simulink model "Pendulo"  (R2018b)
settings: Solver=ode1  StartTime=0.0  StopTime=100.0  FixedStep=0.5  MaxStep=1e-4  RelTol=1e-3
settings Model: Creator=faraday  LastModifiedBy=alejandro

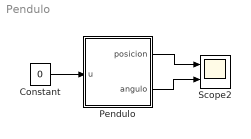
== system Pendulo ==
  Constant : Constant  Value=0
  Pendulo : Subsystem  mask{mc=10, mp=1, l=4, g=9.8, fc=0, fp=0, x10=0, x20=0, x30=pi/2, x40=0}
      mask prompts: mc "masa carro"; mp "masa pendulo"; l "longitud barra"; g "gravedad"; fc "friccion carro"; fp "friccion pendulo"; x10 "posicion inicial"; x20 "velocidad inicial"; x30 "angulo inicial"; x40 "velocidad angular inicial"
  Scope2 : Scope  NumInputPorts=2
  wires:
  Pendulo/1(posicion) -> Scope2/1
  Constant/1 -> Pendulo/1("u ")
  Pendulo/2(angulo) -> Scope2/2

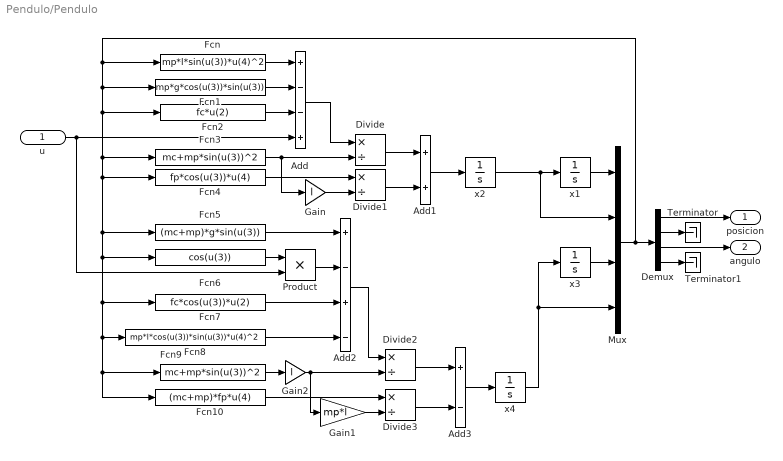
== system Pendulo/Pendulo ==
  "u " : Inport
  Add : Sum  Inputs=+--+
  Add1 : Sum
  Add2 : Sum  Inputs=+-+-
  Add3 : Sum  Inputs=+-
  Demux : Demux
  Divide{,1..3} (4 alike) : Product  Inputs=*/
  Fcn : Fcn  Expr=mp*l*sin(u(3))*u(4)^2
  Fcn1 : Fcn  Expr=mp*g*cos(u(3))*sin(u(3))
  Fcn10 : Fcn  Expr=(mc+mp)*fp*u(4)
  Fcn2 : Fcn  Expr=fc*u(2)
  Fcn3 : Fcn  Expr=mc+mp*sin(u(3))^2
  Fcn4 : Fcn  Expr=fp*cos(u(3))*u(4)
  Fcn5 : Fcn  Expr=(mc+mp)*g*sin(u(3))
  Fcn6 : Fcn  Expr=cos(u(3))
  Fcn7 : Fcn  Expr=fc*cos(u(3))*u(2)
  Fcn8 : Fcn  Expr=mp*l*cos(u(3))*sin(u(3))*u(4)^2
  Fcn9 : Fcn  Expr=mc+mp*sin(u(3))^2
  Gain : Gain  Gain=l
  Gain1 : Gain  Gain=mp*l
  Gain2 : Gain  Gain=l
  Mux : Mux
  Product : Product
  Terminator : Terminator
  Terminator1 : Terminator
  x1 : Integrator  InitialCondition=x10
  x2 : Integrator  InitialCondition=x20
  x3 : Integrator  InitialCondition=x30
  "x4 " : Integrator  InitialCondition=x40
  posicion : Outport
  angulo : Outport  Port=2
  wires:
  Fcn/1 -> Add/1
  Fcn1/1 -> Add/2
  Fcn2/1 -> Add/3
  "u "/1 -> Add/4, Product/2
  Add/1 -> Divide/1
  Fcn3/1 -> Gain/1, Divide/2
  Divide/1 -> Add1/1
  Divide1/1 -> Add1/2
  Add1/1 -> x2/1
  x2/1 -> x1/1, Mux/2
  x1/1 -> Mux/1
  Mux/1 -> Fcn/1, Fcn1/1, Fcn2/1, Fcn3/1, Fcn5/1, Fcn6/1, Fcn10/1, Fcn9/1, Fcn8/1, Fcn7/1, Fcn4/1, Demux/1
  Fcn6/1 -> Product/1
  Product/1 -> Add2/2
  Fcn5/1 -> Add2/1
  Fcn7/1 -> Add2/3
  Fcn8/1 -> Add2/4
  Divide2/1 -> Add3/1
  Add2/1 -> Divide2/1
  Gain/1 -> Divide1/2
  Fcn4/1 -> Divide1/1
  Divide3/1 -> Add3/2
  Fcn10/1 -> Divide3/1
  Gain1/1 -> Divide3/2
  Add3/1 -> "x4 "/1
  "x4 "/1 -> Mux/4, x3/1
  x3/1 -> Mux/3
  Fcn9/1 -> Gain2/1
  Gain2/1 -> Gain1/1, Divide2/2
  Demux/3 -> angulo/1
  Demux/2 -> Terminator/1
  Demux/4 -> Terminator1/1
  Demux/1 -> posicion/1
